simulink model "Quadrotor_Simulink_Model"  (R2019b)
settings: Solver=ode3  StartTime=0.0  StopTime=30  FixedStep=1e-3
values from neighbouring files (symbols this model uses):
  a1 = 2.8    [Main.m]
  a2 = 3.75    [Main.m]
  a3 = a1    (= 2.8)    [Main.m]
  a4 = a2    (= 3.75)    [Main.m]
  a5 = a1    (= 2.8)    [Main.m]
  a6 = a2    (= 3.75)    [Main.m]
  g = 9.81    [Main.m]
  Ix = 0.038    [Main.m]
  Iy = 0.033    [Main.m]
  Iz = 0.079    [Main.m]
  Jr = Iz    (= 0.079)    [Main.m]
  k1 = kd    (= 1e-08)    [Main.m]
  k2 = k1    (= 1e-08)    [Main.m]
  k3 = k1    (= 1e-08)    [Main.m]
  k4 = k1    (= 1e-08)    [Main.m]
  k5 = kpd    (= 4e-07)    [Main.m]
  k6 = k5    (= 4e-07)    [Main.m]
  kd = 1e-8    (= 1e-08)    [Main.m]
  kpt = 8e-6    (= 8e-06)    [Main.m]
  kt = 7e-7    (= 7e-07)    [Main.m]
  l = 12/2/39.37    (= 0.152400304801)    [Main.m]
  lam1 = 15.94    [Main.m]
  lam2 = 52.42    [Main.m]
  lam3 = 15.94    [Main.m]
  lam4 = lam2    (= 52.42)    [Main.m]
  lam5 = 15.94    [Main.m]
  mt = 2.45+1    (= 3.45)    [Main.m]
  omg5pow2 = 3479    [Main.m]
  omg6pow2 = omg5pow2    (= 3479)    [Main.m]
settings Model: Creator=Atiyeh  LastModifiedBy=Atiyeh
settings SolverCC: AlgebraicLoopSolver=LineSearch

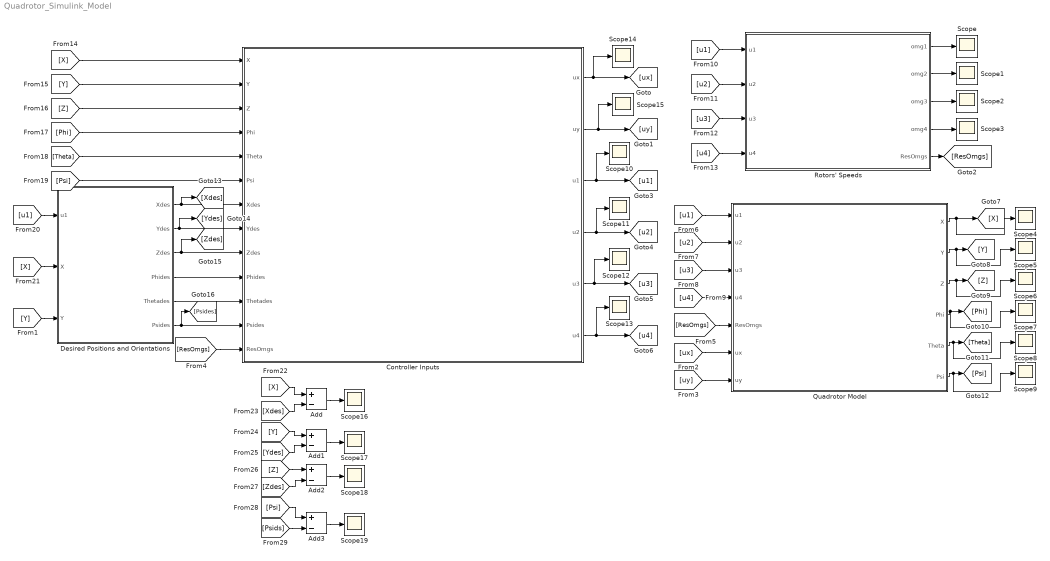
== system Quadrotor_Simulink_Model ==
  Add{,1..3} (4 alike) : Sum  Inputs=+-
  Controller Inputs : Subsystem
  Desired Positions and Orientations : Subsystem
  Quadrotor Model : Subsystem
  Rotors' Speeds : Subsystem
  Scope{,1..19} (20 alike) : Scope
  wires:
  Rotors' Speeds/5(ResOmgs) -> [ResOmgs]
  Desired Positions and Orientations/1("Xdes ") -> [Xdes], Controller Inputs/7(Xdes)
  Desired Positions and Orientations/2(Ydes) -> [Ydes], Controller Inputs/8(Ydes)
  Desired Positions and Orientations/3(Zdes) -> [Zdes], Controller Inputs/9(Zdes)
  Controller Inputs/2("uy ") -> Scope15/1, [uy]
  Controller Inputs/1("ux ") -> Scope14/1, [ux]
  [ResOmgs] -> Controller Inputs/13(ResOmgs)
  [ResOmgs] -> Quadrotor Model/5(ResOmgs)
  Controller Inputs/6("u4   ") -> [u4], Scope13/1
  Controller Inputs/5("u3   ") -> [u3], Scope12/1
  Controller Inputs/3("u1 ") -> Scope10/1, [u1]
  Controller Inputs/4("u2  ") -> [u2], Scope11/1
  [u1] -> Quadrotor Model/1(u1)
  [u2] -> Quadrotor Model/2(u2)
  [u3] -> Quadrotor Model/3(u3)
  [u4] -> Quadrotor Model/4(u4)
  [u2] -> Rotors' Speeds/2(u2)
  [u4] -> Rotors' Speeds/4(u4)
  [u3] -> Rotors' Speeds/3(u3)
  [u1] -> Rotors' Speeds/1(u1)
  Rotors' Speeds/1(omg1) -> Scope/1
  Rotors' Speeds/2(omg2) -> Scope1/1
  Rotors' Speeds/3(omg3) -> Scope2/1
  Rotors' Speeds/4(omg4) -> Scope3/1
  Quadrotor Model/1("X ") -> Scope4/1, [X]
  Quadrotor Model/6("Psi ") -> Scope9/1, [Psi]
  Quadrotor Model/5("Theta ") -> Scope8/1, [Theta]
  Quadrotor Model/4("Phi ") -> Scope7/1, [Phi]
  Quadrotor Model/3("Z ") -> Scope6/1, [Z]
  Quadrotor Model/2("Y ") -> Scope5/1, [Y]
  [X] -> Controller Inputs/1(X)
  [Y] -> Controller Inputs/2(Y)
  [Z] -> Controller Inputs/3(Z)
  [Phi] -> Controller Inputs/4(Phi)
  [Theta] -> Controller Inputs/5(Theta)
  [Psi] -> Controller Inputs/6(Psi)
  [uy] -> Quadrotor Model/7(uy)
  [ux] -> Quadrotor Model/6(ux)
  [u1] -> Desired Positions and Orientations/1(u1)
  [X] -> Desired Positions and Orientations/2(X)
  [Y] -> Desired Positions and Orientations/3(Y)
  Desired Positions and Orientations/4(Phides) -> Controller Inputs/10(Phides)
  Desired Positions and Orientations/6(Psides) -> [Psides], Controller Inputs/12(Psides)
  Desired Positions and Orientations/5(Thetades) -> Controller Inputs/11(Thetades)
  [X] -> Add/1
  [Xdes] -> Add/2
  [Z] -> Add2/1
  [Psids] -> Add3/2
  [Y] -> Add1/1
  [Ydes] -> Add1/2
  [Zdes] -> Add2/2
  [Psi] -> Add3/1
  Add/1 -> Scope16/1
  Add1/1 -> Scope17/1
  Add2/1 -> Scope18/1
  Add3/1 -> Scope19/1

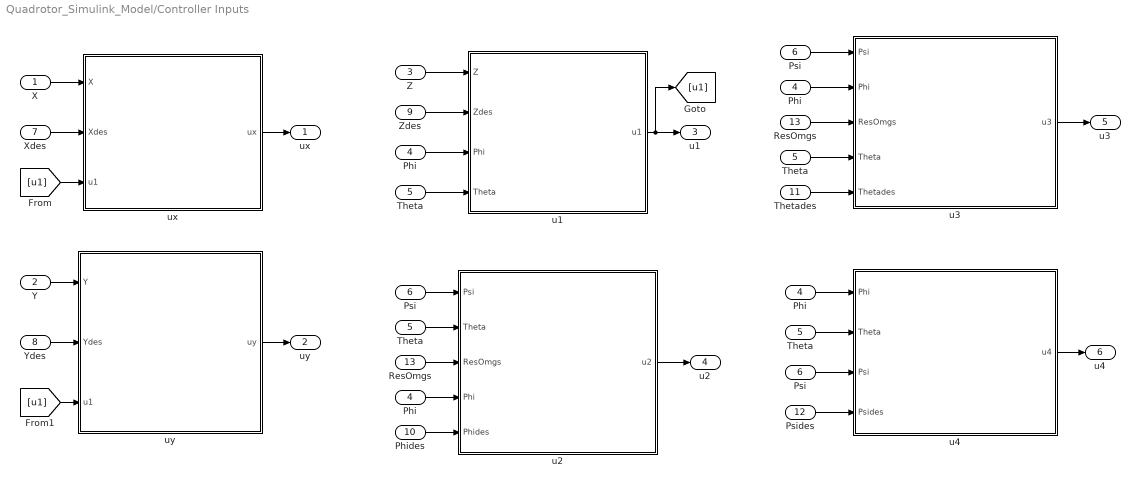
== system Quadrotor_Simulink_Model/Controller Inputs ==
  X : Inport
  Y : Inport  Port=2
  Z : Inport  Port=3
  Phi : Inport  Port=4
  Theta : Inport  Port=5
  Psi : Inport  Port=6
  Xdes : Inport  Port=7
  Ydes : Inport  Port=8
  Zdes : Inport  Port=9
  Phides : Inport  Port=10
  Thetades : Inport  Port=11
  Psides : Inport  Port=12
  ResOmgs : Inport  Port=13
  "Phi " : InportShadow  Port=4
  "Phi  " : InportShadow  Port=4
  "Phi    " : InportShadow  Port=4
  "Psi " : InportShadow  Port=6
  "Psi   " : InportShadow  Port=6
  "ResOmgs " : InportShadow  Port=13
  "Theta " : InportShadow  Port=5
  "Theta  " : InportShadow  Port=5
  "Theta    " : InportShadow  Port=5
  u1 : Subsystem
  "u2 " : Subsystem
  "u3 " : Subsystem
  "u4 " : Subsystem
  ux : Subsystem
  uy : Subsystem
  "ux " : Outport
  "uy " : Outport  Port=2
  "u1 " : Outport  Port=3
  "u2  " : Outport  Port=4
  "u3   " : Outport  Port=5
  "u4   " : Outport  Port=6
  wires:
  ux/1("ux ") -> "ux "/1
  "u2 "/1(u2) -> "u2  "/1
  "u3 "/1(u3) -> "u3   "/1
  "u4 "/1(u4) -> "u4   "/1
  u1/1("u1 ") -> [u1], "u1 "/1
  X/1 -> ux/1(X)
  Xdes/1 -> ux/2(Xdes)
  [u1] -> ux/3(u1)
  Y/1 -> uy/1(Y)
  Phi/1 -> u1/3(Phi)
  Theta/1 -> u1/4(Theta)
  Zdes/1 -> u1/2(Zdes)
  Z/1 -> u1/1(Z)
  Psi/1 -> "u2 "/1(Psi)
  "Theta "/1 -> "u2 "/2(Theta)
  ResOmgs/1 -> "u2 "/3(ResOmgs)
  "Phi "/1 -> "u2 "/4(Phi)
  Phides/1 -> "u2 "/5(Phides)
  "Psi "/1 -> "u3 "/1(Psi)
  "Phi  "/1 -> "u3 "/2("Phi   ")
  "ResOmgs "/1 -> "u3 "/3(ResOmgs)
  "Theta  "/1 -> "u3 "/4(Theta)
  Thetades/1 -> "u3 "/5(Thetades)
  "Phi    "/1 -> "u4 "/1(Phi)
  "Theta    "/1 -> "u4 "/2("Theta    ")
  "Psi   "/1 -> "u4 "/3(Psi)
  Psides/1 -> "u4 "/4(Psides)
  Ydes/1 -> uy/2(Ydes)
  [u1] -> uy/3(u1)
  uy/1("uy ") -> "uy "/1

== system Quadrotor_Simulink_Model/Desired Positions and Orientations ==
  u1 : Inport
  X : Inport  Port=2
  Y : Inport  Port=3
  Phidesired : Subsystem
  Psidesired : Subsystem
  Thetadesired : Subsystem
  Xdesired : Subsystem
  Ydesired : Subsystem
  Zdesired : Subsystem
  "u1 " : InportShadow
  "Xdes " : Outport
  Ydes : Outport  Port=2
  Zdes : Outport  Port=3
  Phides : Outport  Port=4
  Thetades : Outport  Port=5
  Psides : Outport  Port=6
  wires:
  Xdesired/1("Xdes ") -> [Xdes], "Xdes "/1
  Ydesired/1(Ydes) -> [Ydes], Ydes/1
  Zdesired/1(Zdes) -> Zdes/1
  Psidesired/1(Psides) -> Psides/1
  X/1 -> Thetadesired/3(X)
  u1/1 -> Thetadesired/2(u1)
  Y/1 -> Phidesired/3(y)
  "u1 "/1 -> Phidesired/4(u1)
  [Thetades] -> Phidesired/1(Thetades)
  [Xdes] -> Thetadesired/1(xdes)
  Thetadesired/1(Thetades) -> Thetades/1, [Thetades]
  Phidesired/1(Phides) -> Phides/1
  [Ydes] -> Phidesired/2(ydes)

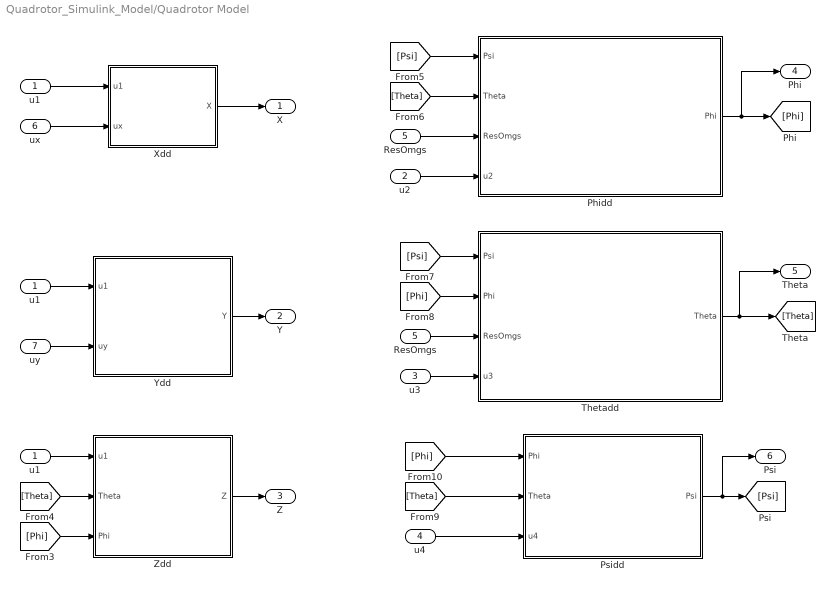
== system Quadrotor_Simulink_Model/Quadrotor Model ==
  u1 : Inport
  u2 : Inport  Port=2
  u3 : Inport  Port=3
  u4 : Inport  Port=4
  ResOmgs : Inport  Port=5
  ux : Inport  Port=6
  uy : Inport  Port=7
  Phidd : Subsystem
  Psidd : Subsystem
  "ResOmgs " : InportShadow  Port=5
  Thetadd : Subsystem
  Xdd : Subsystem
  Ydd : Subsystem
  Zdd : Subsystem
  "u1 " : InportShadow
  "u1  " : InportShadow
  "X " : Outport
  "Y " : Outport  Port=2
  "Z " : Outport  Port=3
  "Phi " : Outport  Port=4
  "Theta " : Outport  Port=5
  "Psi " : Outport  Port=6
  wires:
  "u1 "/1 -> Xdd/1(u1)
  Xdd/1(X) -> "X "/1
  u1/1 -> Zdd/1(u1)
  u4/1 -> Psidd/3(u4)
  u3/1 -> Thetadd/4(u3)
  Phidd/1(Phi) -> [Phi], "Phi "/1
  u2/1 -> Phidd/4(u2)
  ux/1 -> Xdd/2(ux)
  Ydd/1(Y) -> "Y "/1
  Zdd/1(Z) -> "Z "/1
  [Theta] -> Zdd/2(Theta)
  [Phi] -> Zdd/3(Phi)
  [Psi] -> Phidd/1(Psi)
  [Theta] -> Phidd/2(Theta)
  ResOmgs/1 -> Phidd/3(ResOmgs)
  "ResOmgs "/1 -> Thetadd/3(ResOmgs)
  [Psi] -> Thetadd/1(Psi)
  [Phi] -> Thetadd/2("Phi ")
  Thetadd/1(Theta) -> "Theta "/1, [Theta]
  [Theta] -> Psidd/2("Theta ")
  [Phi] -> Psidd/1(Phi)
  Psidd/1(Psi) -> "Psi "/1, [Psi]
  "u1  "/1 -> Ydd/1(u1)
  uy/1 -> Ydd/2(uy)

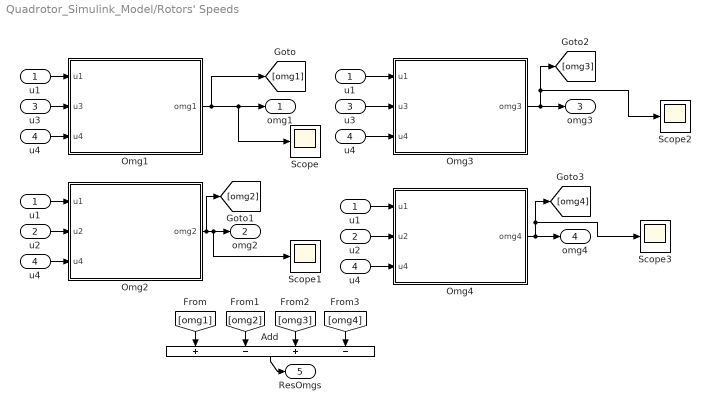
== system Quadrotor_Simulink_Model/Rotors' Speeds ==
  u1 : Inport
  u2 : Inport  Port=2
  u3 : Inport  Port=3
  u4 : Inport  Port=4
  Add : Sum  Inputs=+-+-
  Omg1 : Subsystem
  Omg2 : Subsystem
  Omg3 : Subsystem
  Omg4 : Subsystem
  Scope{,1..3} (4 alike) : Scope
  "u1 " : InportShadow
  "u1  " : InportShadow
  "u1   " : InportShadow
  "u2 " : InportShadow  Port=2
  "u3 " : InportShadow  Port=3
  "u4 " : InportShadow  Port=4
  "u4  " : InportShadow  Port=4
  "u4    " : InportShadow  Port=4
  omg1 : Outport
  omg2 : Outport  Port=2
  omg3 : Outport  Port=3
  omg4 : Outport  Port=4
  ResOmgs : Outport  Port=5
  wires:
  u1/1 -> Omg1/1(u1)
  u4/1 -> Omg1/3(u4)
  Omg1/1(omg1) -> [omg1], Scope/1, omg1/1
  Omg2/1(omg2) -> [omg2], Scope1/1, omg2/1
  "u4 "/1 -> Omg2/3(u4)
  u2/1 -> Omg2/2(u2)
  "u1 "/1 -> Omg2/1(u1)
  Omg4/1(omg4) -> Scope3/1, [omg4], omg4/1
  "u4    "/1 -> Omg4/3(u4)
  "u1   "/1 -> Omg4/1(u1)
  u3/1 -> Omg1/2(u3)
  "u3 "/1 -> Omg3/2(u3)
  Omg3/1(omg3) -> Scope2/1, [omg3], omg3/1
  "u4  "/1 -> Omg3/3(u4)
  "u1  "/1 -> Omg3/1(u1)
  "u2 "/1 -> Omg4/2(u2)
  [omg1] -> Add/1
  [omg2] -> Add/2
  [omg3] -> Add/3
  [omg4] -> Add/4
  Add/1 -> ResOmgs/1

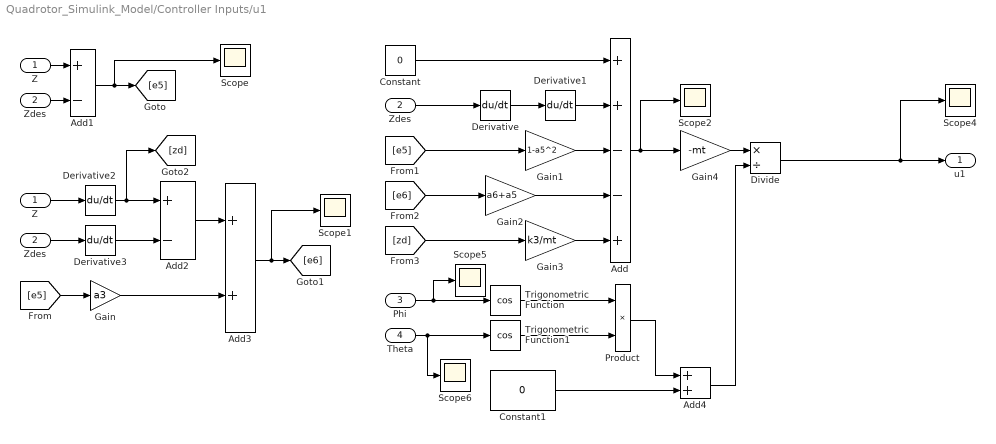
== system Quadrotor_Simulink_Model/Controller Inputs/u1 ==
  Z : Inport
  Zdes : Inport  Port=2
  Phi : Inport  Port=3
  Theta : Inport  Port=4
  Add : Sum  Inputs=++--+
  Add1 : Sum  Inputs=+-
  Add2 : Sum  Inputs=+-
  Add3 : Sum
  Add4 : Sum
  Constant : Constant  Value=0
  Constant1 : Constant  Value=0
  Derivative{,1..3} (4 alike) : Derivative
  Divide : Product  Inputs=*/
  Gain : Gain  Gain=a3
  Gain1 : Gain  Gain=1-a5^2
  Gain2 : Gain  Gain=a6+a5
  Gain3 : Gain  Gain=k3/mt
  Gain4 : Gain  Gain=-mt
  Product : Product
  Scope{,1..2,4..6} (6 alike) : Scope
  Trigonometric Function : Trigonometry  Operator=cos
  Trigonometric Function1 : Trigonometry  Operator=cos
  "Z  " : InportShadow
  "Zdes " : InportShadow  Port=2
  "Zdes  " : InportShadow  Port=2
  "u1 " : Outport
  wires:
  "Z  "/1 -> Derivative2/1
  Phi/1 -> Scope5/1, Trigonometric Function/1
  Gain4/1 -> Divide/1
  [e5] -> Gain1/1
  Gain1/1 -> Add/3
  Z/1 -> Add1/1
  Add/1 -> Scope2/1, Gain4/1
  Gain/1 -> Add3/2
  [zd] -> Gain3/1
  Add2/1 -> Add3/1
  Add1/1 -> Scope/1, [e5]
  Gain3/1 -> Add/5
  [e5] -> Gain/1
  Add3/1 -> Scope1/1, [e6]
  Gain2/1 -> Add/4
  "Zdes "/1 -> Add1/2
  [e6] -> Gain2/1
  Derivative2/1 -> [zd], Add2/1
  "Zdes  "/1 -> Derivative3/1
  Derivative3/1 -> Add2/2
  Derivative1/1 -> Add/2
  Derivative/1 -> Derivative1/1
  Zdes/1 -> Derivative/1
  Constant/1 -> Add/1
  Theta/1 -> Scope6/1, Trigonometric Function1/1
  Trigonometric Function/1 -> Product/1
  Trigonometric Function1/1 -> Product/2
  Product/1 -> Add4/1
  Constant1/1 -> Add4/2
  Divide/1 -> "u1 "/1, Scope4/1
  Add4/1 -> Divide/2

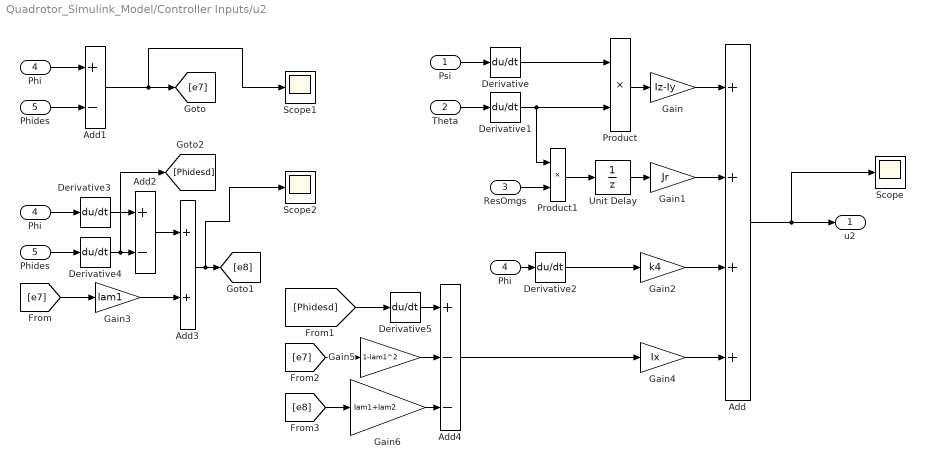
== system Quadrotor_Simulink_Model/Controller Inputs/u2  ==
  Psi : Inport
  Theta : Inport  Port=2
  ResOmgs : Inport  Port=3
  Phi : Inport  Port=4
  Phides : Inport  Port=5
  Add : Sum  Inputs=++++
  Add1 : Sum  Inputs=+-
  Add2 : Sum  Inputs=+-
  Add3 : Sum
  Add4 : Sum  Inputs=+--
  Derivative{,1..5} (6 alike) : Derivative
  Gain : Gain  Gain=Iz-Iy
  Gain1 : Gain  Gain=Jr
  Gain2 : Gain  Gain=k4
  Gain3 : Gain  Gain=lam1
  Gain4 : Gain  Gain=Ix
  Gain5 : Gain  Gain=1-lam1^2
  Gain6 : Gain  Gain=lam1+lam2
  "Phi " : InportShadow  Port=4
  "Phi  " : InportShadow  Port=4
  "Phides " : InportShadow  Port=5
  Product : Product
  Product1 : Product
  Scope : Scope
  Scope1 : Scope
  Scope2 : Scope
  Unit Delay : UnitDelay  SampleTime=-1  HasFrameUpgradeWarning=on
  u2 : Outport
  wires:
  Psi/1 -> Derivative/1
  Theta/1 -> Derivative1/1
  Derivative/1 -> Product/1
  Product/1 -> Gain/1
  Gain/1 -> Add/1
  ResOmgs/1 -> Product1/2
  Product1/1 -> Unit Delay/1
  Gain1/1 -> Add/2
  Gain2/1 -> Add/3
  Phi/1 -> Derivative2/1
  Derivative2/1 -> Gain2/1
  "Phi "/1 -> Add1/1
  Phides/1 -> Add1/2
  Add1/1 -> Scope1/1, [e7]
  "Phides "/1 -> Derivative4/1
  "Phi  "/1 -> Derivative3/1
  Derivative3/1 -> Add2/1
  Derivative4/1 -> [Phidesd], Add2/2
  [e7] -> Gain3/1
  Add2/1 -> Add3/1
  Gain3/1 -> Add3/2
  Add3/1 -> Scope2/1, [e8]
  [Phidesd] -> Derivative5/1
  Derivative5/1 -> Add4/1
  Gain4/1 -> Add/4
  Gain5/1 -> Add4/2
  [e7] -> Gain5/1
  Gain6/1 -> Add4/3
  [e8] -> Gain6/1
  Add4/1 -> Gain4/1
  Add/1 -> Scope/1, u2/1
  Derivative1/1 -> Product1/1, Product/2
  Unit Delay/1 -> Gain1/1

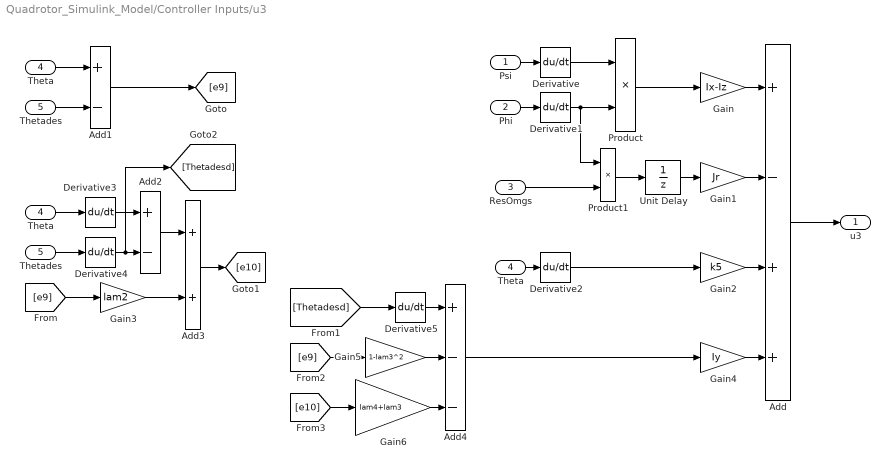
== system Quadrotor_Simulink_Model/Controller Inputs/u3  ==
  Psi : Inport
  "Phi   " : Inport  Port=2
  ResOmgs : Inport  Port=3
  Theta : Inport  Port=4
  Thetades : Inport  Port=5
  Add : Sum  Inputs=+-++
  Add1 : Sum  Inputs=+-
  Add2 : Sum  Inputs=+-
  Add3 : Sum
  Add4 : Sum  Inputs=+--
  Derivative{,1..5} (6 alike) : Derivative
  Gain : Gain  Gain=Ix-Iz
  Gain1 : Gain  Gain=Jr
  Gain2 : Gain  Gain=k5
  Gain3 : Gain  Gain=lam2
  Gain4 : Gain  Gain=Iy
  Gain5 : Gain  Gain=1-lam3^2
  Gain6 : Gain  Gain=lam4+lam3
  Product : Product
  Product1 : Product
  "Theta " : InportShadow  Port=4
  "Theta   " : InportShadow  Port=4
  "Thetades  " : InportShadow  Port=5
  Unit Delay : UnitDelay  SampleTime=-1  HasFrameUpgradeWarning=on
  u3 : Outport
  wires:
  "Theta "/1 -> Add1/1
  Add3/1 -> [e10]
  Derivative1/1 -> Product1/1, Product/2
  Thetades/1 -> Add1/2
  Gain4/1 -> Add/4
  "Phi   "/1 -> Derivative1/1
  Gain/1 -> Add/1
  "Thetades  "/1 -> Derivative4/1
  [e9] -> Gain5/1
  Gain3/1 -> Add3/2
  [Thetadesd] -> Derivative5/1
  Product/1 -> Gain/1
  Gain2/1 -> Add/3
  Psi/1 -> Derivative/1
  Add1/1 -> [e9]
  Derivative4/1 -> [Thetadesd], Add2/2
  [e9] -> Gain3/1
  Add4/1 -> Gain4/1
  Add2/1 -> Add3/1
  Theta/1 -> Derivative2/1
  [e10] -> Gain6/1
  Gain5/1 -> Add4/2
  Gain6/1 -> Add4/3
  Derivative2/1 -> Gain2/1
  "Theta   "/1 -> Derivative3/1
  Derivative5/1 -> Add4/1
  Gain1/1 -> Add/2
  Derivative/1 -> Product/1
  Derivative3/1 -> Add2/1
  Add/1 -> u3/1
  Product1/1 -> Unit Delay/1
  ResOmgs/1 -> Product1/2
  Unit Delay/1 -> Gain1/1

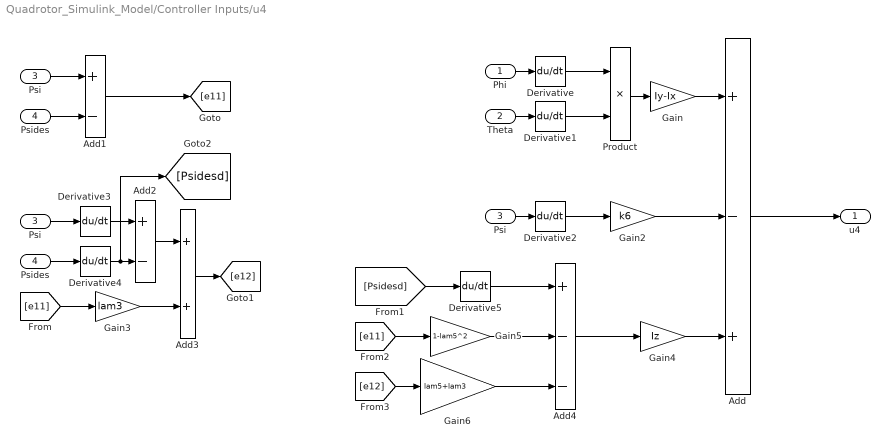
== system Quadrotor_Simulink_Model/Controller Inputs/u4  ==
  Phi : Inport
  "Theta    " : Inport  Port=2
  Psi : Inport  Port=3
  Psides : Inport  Port=4
  Add : Sum  Inputs=+-+
  Add1 : Sum  Inputs=+-
  Add2 : Sum  Inputs=+-
  Add3 : Sum
  Add4 : Sum  Inputs=+--
  Derivative{,1..5} (6 alike) : Derivative
  Gain : Gain  Gain=Iy-Ix
  Gain2 : Gain  Gain=k6
  Gain3 : Gain  Gain=lam3
  Gain4 : Gain  Gain=Iz
  Gain5 : Gain  Gain=1-lam5^2
  Gain6 : Gain  Gain=lam5+lam3
  Product : Product
  "Psi  " : InportShadow  Port=3
  "Psi     " : InportShadow  Port=3
  "Psides    " : InportShadow  Port=4
  u4 : Outport
  wires:
  Product/1 -> Gain/1
  Gain2/1 -> Add/2
  Phi/1 -> Derivative/1
  [Psidesd] -> Derivative5/1
  [e11] -> Gain5/1
  Gain3/1 -> Add3/2
  Gain/1 -> Add/1
  "Theta    "/1 -> Derivative1/1
  Derivative1/1 -> Product/2
  Add/1 -> u4/1
  Add3/1 -> [e12]
  Derivative3/1 -> Add2/1
  Psides/1 -> Add1/2
  Derivative/1 -> Product/1
  "Psi     "/1 -> Derivative3/1
  "Psi  "/1 -> Add1/1
  Derivative5/1 -> Add4/1
  Derivative2/1 -> Gain2/1
  Gain6/1 -> Add4/3
  Gain5/1 -> Add4/2
  [e12] -> Gain6/1
  Add2/1 -> Add3/1
  Add4/1 -> Gain4/1
  [e11] -> Gain3/1
  Psi/1 -> Derivative2/1
  Gain4/1 -> Add/3
  Add1/1 -> [e11]
  "Psides    "/1 -> Derivative4/1
  Derivative4/1 -> [Psidesd], Add2/2

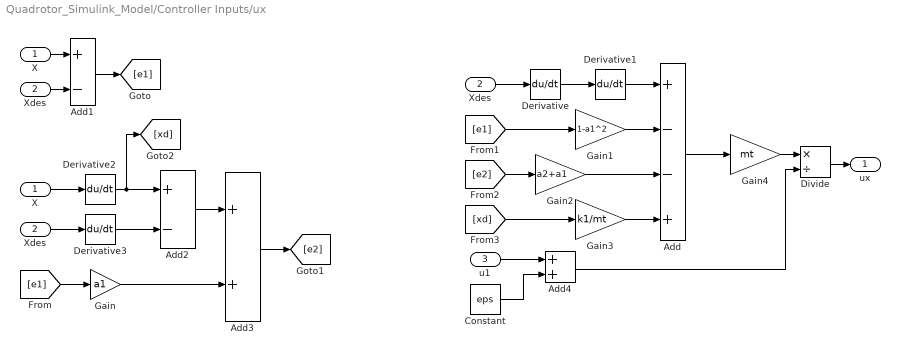
== system Quadrotor_Simulink_Model/Controller Inputs/ux ==
  X : Inport
  Xdes : Inport  Port=2
  u1 : Inport  Port=3
  Add : Sum  Inputs=+--+
  Add1 : Sum  Inputs=+-
  Add2 : Sum  Inputs=+-
  Add3 : Sum
  Add4 : Sum
  Constant : Constant  Value=eps
  Derivative{,1..3} (4 alike) : Derivative
  Divide : Product  Inputs=*/
  Gain : Gain  Gain=a1
  Gain1 : Gain  Gain=1-a1^2
  Gain2 : Gain  Gain=a2+a1
  Gain3 : Gain  Gain=k1/mt
  Gain4 : Gain  Gain=mt
  "X  " : InportShadow
  "Xdes " : InportShadow  Port=2
  "Xdes  " : InportShadow  Port=2
  "ux " : Outport
  wires:
  Derivative/1 -> Derivative1/1
  Xdes/1 -> Derivative/1
  Derivative1/1 -> Add/1
  "X  "/1 -> Derivative2/1
  "Xdes  "/1 -> Derivative3/1
  Derivative2/1 -> [xd], Add2/1
  Derivative3/1 -> Add2/2
  Add2/1 -> Add3/1
  [e1] -> Gain/1
  Gain/1 -> Add3/2
  Add3/1 -> [e2]
  [e1] -> Gain1/1
  Gain1/1 -> Add/2
  Add1/1 -> [e1]
  X/1 -> Add1/1
  "Xdes "/1 -> Add1/2
  [e2] -> Gain2/1
  Gain2/1 -> Add/3
  [xd] -> Gain3/1
  Gain3/1 -> Add/4
  Add/1 -> Gain4/1
  Gain4/1 -> Divide/1
  Divide/1 -> "ux "/1
  u1/1 -> Add4/1
  Constant/1 -> Add4/2
  Add4/1 -> Divide/2

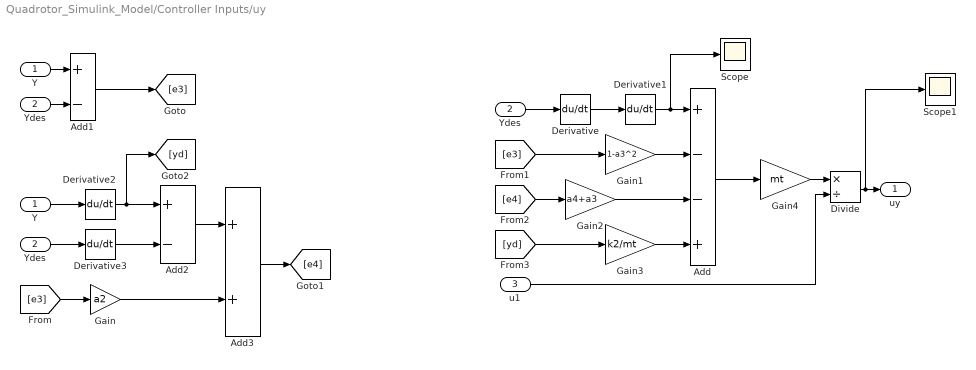
== system Quadrotor_Simulink_Model/Controller Inputs/uy ==
  Y : Inport
  Ydes : Inport  Port=2
  u1 : Inport  Port=3
  Add : Sum  Inputs=+--+
  Add1 : Sum  Inputs=+-
  Add2 : Sum  Inputs=+-
  Add3 : Sum
  Derivative{,1..3} (4 alike) : Derivative
  Divide : Product  Inputs=*/
  Gain : Gain  Gain=a2
  Gain1 : Gain  Gain=1-a3^2
  Gain2 : Gain  Gain=a4+a3
  Gain3 : Gain  Gain=k2/mt
  Gain4 : Gain  Gain=mt
  Scope : Scope
  Scope1 : Scope
  "Y   " : InportShadow
  "Ydes " : InportShadow  Port=2
  "Ydes   " : InportShadow  Port=2
  "uy " : Outport
  wires:
  "Y   "/1 -> Derivative2/1
  u1/1 -> Divide/2
  Gain4/1 -> Divide/1
  [e3] -> Gain1/1
  Gain1/1 -> Add/2
  Y/1 -> Add1/1
  Add/1 -> Gain4/1
  Gain/1 -> Add3/2
  [yd] -> Gain3/1
  Add2/1 -> Add3/1
  Add1/1 -> [e3]
  Gain3/1 -> Add/4
  [e3] -> Gain/1
  Add3/1 -> [e4]
  Gain2/1 -> Add/3
  "Ydes "/1 -> Add1/2
  [e4] -> Gain2/1
  Derivative2/1 -> [yd], Add2/1
  "Ydes   "/1 -> Derivative3/1
  Derivative3/1 -> Add2/2
  Derivative1/1 -> Scope/1, Add/1
  Derivative/1 -> Derivative1/1
  Ydes/1 -> Derivative/1
  Divide/1 -> Scope1/1, "uy "/1

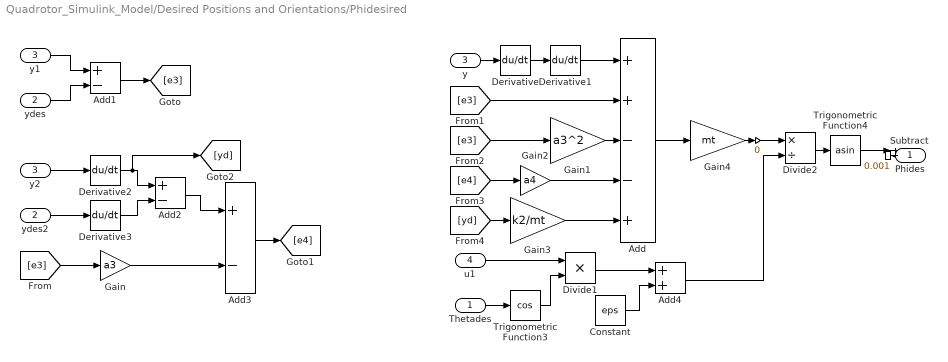
== system Quadrotor_Simulink_Model/Desired Positions and Orientations/Phidesired ==
  Thetades : Inport
  ydes : Inport  Port=2
  y : Inport  Port=3
  u1 : Inport  Port=4
  " " : Gain  Gain=0
  "  " : Constant  Value=0.001
  Add : Sum  Inputs=++--+
  Add1 : Sum  Inputs=+-
  Add2 : Sum  Inputs=+-
  Add3 : Sum  Inputs=+-
  Add4 : Sum
  Constant : Constant  Value=eps
  Derivative{,1..3} (4 alike) : Derivative
  Divide1 : Product  Inputs=**
  Divide2 : Product  Inputs=*/
  Gain : Gain  Gain=a3
  Gain1 : Gain  Gain=a3^2
  Gain2 : Gain  Gain=a4
  Gain3 : Gain  Gain=k2/mt
  Gain4 : Gain  Gain=mt
  Subtract : Sum  Inputs=+-
  Trigonometric Function3 : Trigonometry  Operator=cos
  Trigonometric Function4 : Trigonometry  Operator=asin
  y1 : InportShadow  Port=3
  y2 : InportShadow  Port=3
  ydes2 : InportShadow  Port=2
  Phides : Outport
  wires:
  y/1 -> Derivative/1
  Derivative/1 -> Derivative1/1
  Derivative1/1 -> Add/1
  y1/1 -> Add1/1
  ydes/1 -> Add1/2
  Add1/1 -> [e3]
  y2/1 -> Derivative2/1
  ydes2/1 -> Derivative3/1
  Derivative2/1 -> [yd], Add2/1
  Derivative3/1 -> Add2/2
  Add2/1 -> Add3/1
  [e3] -> Gain/1
  Gain/1 -> Add3/2
  Add3/1 -> [e4]
  [e3] -> Add/2
  [e3] -> Gain1/1
  Gain1/1 -> Add/3
  [e4] -> Gain2/1
  Gain2/1 -> Add/4
  [yd] -> Gain3/1
  Gain3/1 -> Add/5
  Add/1 -> Gain4/1
  u1/1 -> Divide1/1
  Thetades/1 -> Trigonometric Function3/1
  Trigonometric Function3/1 -> Divide1/2
  Divide2/1 -> Trigonometric Function4/1
  Divide1/1 -> Add4/1
  Add4/1 -> Divide2/2
  Constant/1 -> Add4/2
  Gain4/1 -> " "/1
  " "/1 -> Divide2/1
  Subtract/1 -> Phides/1
  Trigonometric Function4/1 -> Subtract/1
  "  "/1 -> Subtract/2

== system Quadrotor_Simulink_Model/Desired Positions and Orientations/Psidesired ==
  Step : Step  Time=0  After=0  SampleTime=0
  Psides : Outport
  wires:
  Step/1 -> Psides/1

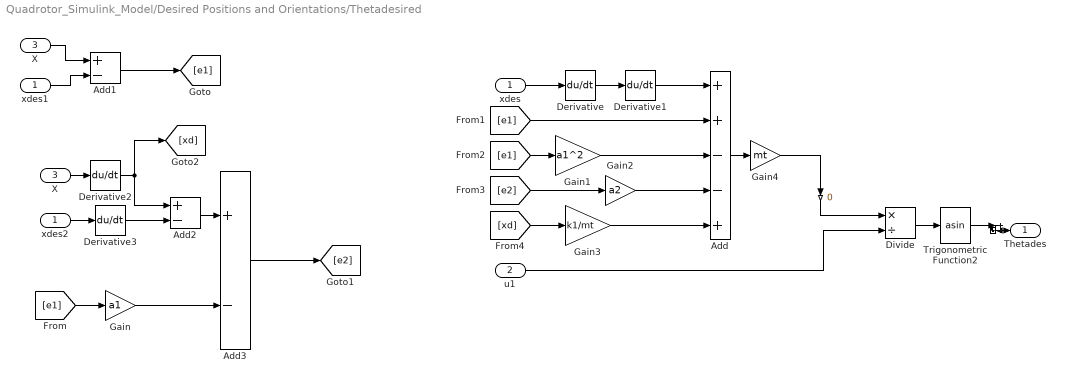
== system Quadrotor_Simulink_Model/Desired Positions and Orientations/Thetadesired ==
  xdes : Inport
  u1 : Inport  Port=2
  X : Inport  Port=3
  " " : Gain  Gain=0
  "  " : Sum
  "   " : Sin  Amplitude=0.001  SampleTime=0
  Add : Sum  Inputs=++--+
  Add1 : Sum  Inputs=+-
  Add2 : Sum  Inputs=+-
  Add3 : Sum  Inputs=+-
  Derivative{,1..3} (4 alike) : Derivative
  Divide : Product  Inputs=*/
  Gain : Gain  Gain=a1
  Gain1 : Gain  Gain=a1^2
  Gain2 : Gain  Gain=a2
  Gain3 : Gain  Gain=k1/mt
  Gain4 : Gain  Gain=mt
  Trigonometric Function2 : Trigonometry  Operator=asin
  "X " : InportShadow  Port=3
  xdes1 : InportShadow
  xdes2 : InportShadow
  Thetades : Outport
  wires:
  xdes/1 -> Derivative/1
  Derivative/1 -> Derivative1/1
  Derivative1/1 -> Add/1
  X/1 -> Add1/1
  xdes1/1 -> Add1/2
  Add1/1 -> [e1]
  "X "/1 -> Derivative2/1
  xdes2/1 -> Derivative3/1
  Derivative2/1 -> Add2/1, [xd]
  Derivative3/1 -> Add2/2
  [e1] -> Gain/1
  Add2/1 -> Add3/1
  Gain/1 -> Add3/2
  Add3/1 -> [e2]
  [e1] -> Add/2
  [e1] -> Gain1/1
  Gain1/1 -> Add/3
  [e2] -> Gain2/1
  Gain2/1 -> Add/4
  [xd] -> Gain3/1
  Gain3/1 -> Add/5
  Add/1 -> Gain4/1
  Gain4/1 -> " "/1
  Divide/1 -> Trigonometric Function2/1
  u1/1 -> Divide/2
  " "/1 -> Divide/1
  "   "/1 -> "  "/2
  Trigonometric Function2/1 -> "  "/1
  "  "/1 -> Thetades/1

== system Quadrotor_Simulink_Model/Desired Positions and Orientations/Xdesired ==
  Gain : Gain  Gain=2
  Sine Wave : Sin  SampleTime=0
  "Xdes " : Outport
  wires:
  Gain/1 -> "Xdes "/1
  Sine Wave/1 -> Gain/1

== system Quadrotor_Simulink_Model/Desired Positions and Orientations/Ydesired ==
  Constant1 : Constant
  Derivative : Derivative
  Derivative1 : Derivative
  Scope : Scope
  Scope1 : Scope
  Step1 : Step  Time=0  SampleTime=0
  Ydes : Outport
  wires:
  Step1/1 -> Derivative1/1, Ydes/1
  Derivative1/1 -> Scope/1, Derivative/1
  Derivative/1 -> Scope1/1

== system Quadrotor_Simulink_Model/Desired Positions and Orientations/Zdesired ==
  Add : Sum
  Constant1 : Constant  Value=2
  Gain1 : Gain  Gain=2
  Sine Wave1 : Sin  Phase=pi/2  SampleTime=0
  Zdes : Outport
  wires:
  Sine Wave1/1 -> Gain1/1
  Add/1 -> Zdes/1
  Constant1/1 -> Add/2
  Gain1/1 -> Add/1

== system Quadrotor_Simulink_Model/Quadrotor Model/Phidd ==
  note: Phi
  note: Phid
  note: Phidd
  Psi : Inport
  Theta : Inport  Port=2
  ResOmgs : Inport  Port=3
  u2 : Inport  Port=4
  Add : Sum  Inputs=+--+
  Derivative : Derivative
  Derivative1 : Derivative
  Gain : Gain  Gain=Iy-Iz
  Gain1 : Gain  Gain=Jr
  Gain2 : Gain  Gain=1/Ix
  Gain3 : Gain  Gain=k4
  Integrator2 : Integrator
  Integrator3 : Integrator
  Product : Product
  Product1 : Product
  Scope : Scope
  Scope1 : Scope
  Phi : Outport
  wires:
  Psi/1 -> Derivative/1
  Theta/1 -> Derivative1/1
  Derivative/1 -> Product/1
  Derivative1/1 -> Product1/1, Product/2
  Product/1 -> Gain/1
  Gain/1 -> Add/1
  Product1/1 -> Gain1/1
  ResOmgs/1 -> Product1/2
  Gain1/1 -> Scope1/1, Add/2
  u2/1 -> Add/4
  Add/1 -> Scope/1, Gain2/1
  Gain2/1 -> Integrator3/1
  Integrator3/1 -> Gain3/1, Integrator2/1
  Integrator2/1 -> Phi/1
  Gain3/1 -> Add/3

== system Quadrotor_Simulink_Model/Quadrotor Model/Psidd ==
  note: Psi
  note: Psid
  note: Psidd
  Phi : Inport
  "Theta " : Inport  Port=2
  u4 : Inport  Port=3
  Add : Sum  Inputs=+-+
  Derivative : Derivative
  Derivative1 : Derivative
  Gain1 : Gain  Gain=Ix-Iy
  Gain3 : Gain  Gain=1/Iz
  Gain4 : Gain  Gain=k6
  Integrator2 : Integrator
  Integrator3 : Integrator
  Product : Product
  Psi : Outport
  wires:
  Gain1/1 -> Add/1
  u4/1 -> Add/3
  Add/1 -> Gain3/1
  "Theta "/1 -> Derivative1/1
  Derivative/1 -> Product/1
  Product/1 -> Gain1/1
  Derivative1/1 -> Product/2
  Gain3/1 -> Integrator3/1
  Phi/1 -> Derivative/1
  Gain4/1 -> Add/2
  Integrator3/1 -> Gain4/1, Integrator2/1
  Integrator2/1 -> Psi/1

== system Quadrotor_Simulink_Model/Quadrotor Model/Thetadd ==
  note: Theta
  note: Thetadd
  note: Thetad
  Psi : Inport
  "Phi " : Inport  Port=2
  ResOmgs : Inport  Port=3
  u3 : Inport  Port=4
  Add : Sum  Inputs=++-+
  Derivative : Derivative
  Derivative1 : Derivative
  Gain1 : Gain  Gain=Iz-Ix
  Gain2 : Gain  Gain=Jr
  Gain3 : Gain  Gain=1/Iy
  Gain4 : Gain  Gain=k5
  Integrator2 : Integrator
  Integrator3 : Integrator
  Product : Product
  Product1 : Product
  Theta : Outport
  wires:
  Integrator2/1 -> Theta/1
  Gain4/1 -> Add/3
  Product1/1 -> Gain2/1
  Psi/1 -> Derivative/1
  Derivative1/1 -> Product1/1, Product/2
  Gain2/1 -> Add/2
  Product/1 -> Gain1/1
  Gain3/1 -> Integrator3/1
  Derivative/1 -> Product/1
  ResOmgs/1 -> Product1/2
  Integrator3/1 -> Gain4/1, Integrator2/1
  "Phi "/1 -> Derivative1/1
  Add/1 -> Gain3/1
  u3/1 -> Add/4
  Gain1/1 -> Add/1

== system Quadrotor_Simulink_Model/Quadrotor Model/Xdd ==
  note: Xdd
  note: X
  note: Xd
  u1 : Inport
  ux : Inport  Port=2
  Gain : Gain  Gain=k1
  Gain1 : Gain  Gain=1/mt
  Integrator : Integrator
  Integrator1 : Integrator
  Product : Product
  Subtract : Sum  Inputs=+-
  X : Outport
  wires:
  u1/1 -> Product/1
  Product/1 -> Subtract/1
  Integrator/1 -> Gain/1, Integrator1/1
  Integrator1/1 -> X/1
  Gain/1 -> Subtract/2
  Subtract/1 -> Gain1/1
  Gain1/1 -> Integrator/1
  ux/1 -> Product/2

== system Quadrotor_Simulink_Model/Quadrotor Model/Ydd ==
  note: Y
  note: Yd
  note: Ydd
  u1 : Inport
  uy : Inport  Port=2
  Add : Sum
  Gain : Gain  Gain=k2
  Gain1 : Gain  Gain=1/mt
  Integrator : Integrator
  Integrator1 : Integrator
  Product : Product
  Trigonometric Function1 : Trigonometry
  Trigonometric Function4 : Trigonometry  Operator=cos
  Y : Outport
  wires:
  Add/1 -> Gain1/1
  Gain1/1 -> Integrator/1
  Integrator/1 -> Gain/1, Integrator1/1
  Integrator1/1 -> Y/1
  Gain/1 -> Add/2
  u1/1 -> Product/1
  Product/1 -> Add/1
  uy/1 -> Product/2

== system Quadrotor_Simulink_Model/Quadrotor Model/Zdd ==
  note: Z
  note: Zd
  note: Zdd
  u1 : Inport
  Theta : Inport  Port=2
  Phi : Inport  Port=3
  Add : Sum  Inputs=++-
  Constant : Constant  Value=mt*g
  Gain : Gain  Gain=k3
  Gain1 : Gain  Gain=1/mt
  Gain2 : Gain  Gain=-1
  Integrator : Integrator
  Integrator1 : Integrator
  Product : Product  Inputs=3
  Trigonometric Function : Trigonometry  Operator=cos
  Trigonometric Function1 : Trigonometry  Operator=cos
  Z : Outport
  wires:
  u1/1 -> Gain2/1
  Phi/1 -> Trigonometric Function/1
  Gain1/1 -> Integrator/1
  Product/1 -> Add/2
  Integrator1/1 -> Z/1
  Add/1 -> Gain1/1
  Integrator/1 -> Gain/1, Integrator1/1
  Theta/1 -> Trigonometric Function1/1
  Gain/1 -> Add/3
  Gain2/1 -> Product/1
  Constant/1 -> Add/1
  Trigonometric Function1/1 -> Product/2
  Trigonometric Function/1 -> Product/3

== system Quadrotor_Simulink_Model/Rotors' Speeds/Omg1 ==
  u1 : Inport
  u3 : Inport  Port=2
  u4 : Inport  Port=3
  Abs2 : Abs
  Add1 : Sum  Inputs=+-
  Add2 : Sum  Inputs=+--
  Constant : Constant  Value=omg5pow2+omg6pow2
  Gain2 : Gain  Gain=kpt
  Gain3 : Gain  Gain=1/(4*kt)
  Gain4 : Gain  Gain=1/(2*l*kt)
  Gain5 : Gain  Gain=1/(4*kd)
  Scope{,1..3} (4 alike) : Scope
  Sqrt2 : Sqrt  SaturateOnIntegerOverflow=on
  omg1 : Outport
  wires:
  u1/1 -> Add1/1
  Constant/1 -> Gain2/1
  Gain2/1 -> Add1/2
  Add1/1 -> Gain3/1
  Gain3/1 -> Scope1/1, Add2/1
  u3/1 -> Gain4/1
  Gain4/1 -> Scope2/1, Add2/2
  u4/1 -> Gain5/1
  Gain5/1 -> Add2/3, Scope3/1
  Add2/1 -> Abs2/1
  Abs2/1 -> Sqrt2/1
  Sqrt2/1 -> Scope/1, omg1/1

== system Quadrotor_Simulink_Model/Rotors' Speeds/Omg2 ==
  u1 : Inport
  u2 : Inport  Port=2
  u4 : Inport  Port=3
  Abs2 : Abs
  Add1 : Sum  Inputs=+-
  Add2 : Sum  Inputs=+-+
  Constant : Constant  Value=omg5pow2+omg6pow2
  Gain2 : Gain  Gain=kpt
  Gain3 : Gain  Gain=1/(4*kt)
  Gain4 : Gain  Gain=1/(2*l*kt)
  Gain5 : Gain  Gain=1/(4*kd)
  Sqrt2 : Sqrt  SaturateOnIntegerOverflow=on
  omg2 : Outport
  wires:
  Gain5/1 -> Add2/3
  u2/1 -> Gain4/1
  Gain2/1 -> Add1/2
  Gain3/1 -> Add2/1
  Gain4/1 -> Add2/2
  u4/1 -> Gain5/1
  Add1/1 -> Gain3/1
  u1/1 -> Add1/1
  Constant/1 -> Gain2/1
  Add2/1 -> Abs2/1
  Abs2/1 -> Sqrt2/1
  Sqrt2/1 -> omg2/1

== system Quadrotor_Simulink_Model/Rotors' Speeds/Omg3 ==
  u1 : Inport
  u3 : Inport  Port=2
  u4 : Inport  Port=3
  Abs2 : Abs
  Add1 : Sum  Inputs=+-
  Add2 : Sum  Inputs=++-
  Constant : Constant  Value=omg5pow2+omg6pow2
  Gain2 : Gain  Gain=kpt
  Gain3 : Gain  Gain=1/(4*kt)
  Gain4 : Gain  Gain=1/(2*l*kt)
  Gain5 : Gain  Gain=1/(4*kd)
  Sqrt2 : Sqrt  SaturateOnIntegerOverflow=on
  Unit Delay : UnitDelay  SampleTime=-1  HasFrameUpgradeWarning=on
  omg3 : Outport
  wires:
  Gain5/1 -> Add2/3
  u4/1 -> Gain5/1
  Gain4/1 -> Add2/2
  u3/1 -> Unit Delay/1
  Gain3/1 -> Add2/1
  Add1/1 -> Gain3/1
  Gain2/1 -> Add1/2
  Constant/1 -> Gain2/1
  u1/1 -> Add1/1
  Unit Delay/1 -> Gain4/1
  Add2/1 -> Abs2/1
  Abs2/1 -> Sqrt2/1
  Sqrt2/1 -> omg3/1

== system Quadrotor_Simulink_Model/Rotors' Speeds/Omg4 ==
  u1 : Inport
  u2 : Inport  Port=2
  u4 : Inport  Port=3
  Abs2 : Abs
  Add1 : Sum  Inputs=+-
  Add2 : Sum  Inputs=+++
  Constant : Constant  Value=omg5pow2+omg6pow2
  Gain2 : Gain  Gain=kpt
  Gain3 : Gain  Gain=1/(4*kt)
  Gain4 : Gain  Gain=1/(2*l*kt)
  Gain5 : Gain  Gain=1/(4*kd)
  Sqrt2 : Sqrt  SaturateOnIntegerOverflow=on
  Unit Delay : UnitDelay  SampleTime=-1  HasFrameUpgradeWarning=on
  omg4 : Outport
  wires:
  u1/1 -> Add1/1
  Add1/1 -> Gain3/1
  Gain2/1 -> Add1/2
  Constant/1 -> Gain2/1
  u2/1 -> Unit Delay/1
  u4/1 -> Gain5/1
  Gain3/1 -> Add2/1
  Gain5/1 -> Add2/3
  Gain4/1 -> Add2/2
  Unit Delay/1 -> Gain4/1
  Add2/1 -> Abs2/1
  Abs2/1 -> Sqrt2/1
  Sqrt2/1 -> omg4/1
